simulink library "Dequiv"  (Simulink 3.00)
settings Model: LastModifiedBy=campa

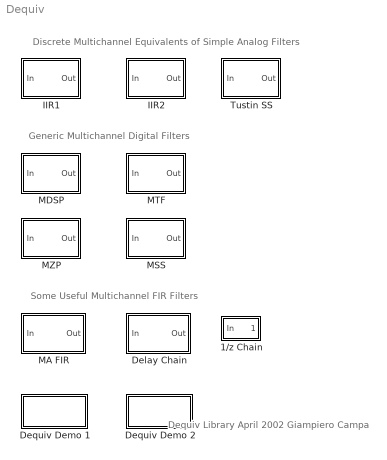
== system Dequiv ==
  note: Discrete Multichannel Equivalents of Simple Analog Filters
  note: Some Useful Multichannel FIR Filters
  note: Dequiv Library
      | April 2002
      | Giampiero Campa
  note: Generic Multichannel Digital Filters
  1/z Chain : Subsystem  mask(Discrete Time FIFO Chain){ni=1, rd=4, x0=0, T=0.025}
      mask prompts: ni "Number of Channels"; rd "Number of Delays for each Channel"; x0 "Initial Conditon"; T "Sample Time"
      mask help: Discrete Time FIFO Chain
      mask init:
      | a=[];b=[];c=[];d=[];
      | for i=1:ni,
      | a=[a,zeros(size(a,1),rd);zeros(rd,size(a,2)),diag(ones(rd-1,1),1)];
      | b=[b,zeros(size(b,1),1);zeros(rd,size(b,2)),[zeros(rd-1,1);1]];
      | c=[c,zeros(size(c,1),rd);zeros(1,size(c,2)),[1 zeros(1,rd-1)]];
      | d=[d,zeros(size(d,1),1);zeros(1,size(d,2)),0];
      | end
      mask Help: Discrete Time FIFO Chain
      mask Display: disp('FIFO')
  Delay Chain : Subsystem  mask(Delay Chain){ni=1, rd=3, x0=2e-7/4, T=0.025}
      mask prompts: ni "Number of Channels"; rd "Number of Delays"; x0 "Initial Condition"; T "Sample Time"
      mask help:
      | Implements a delay chain,
      |   each input is delayed n times and the respective
      |   outputs are all the states as well as the input itself.
      mask init:
      | a=[];b=[];c=[];d=[];
      | for i=1:ni,
      | a=[a,zeros(size(a,1),rd);zeros(rd,size(a,2)),diag(ones(rd-1,1),1)];
      | b=[b,zeros(size(b,1),1);zeros(rd,size(b,2)),[zeros(rd-1,1);1]];
      | c=[c,zeros(size(c,1),rd);zeros(rd+1,size(c,2)),[eye(rd);zeros(1,rd)]];
      | d=[d,zeros(size(d,1),1);zeros(rd+1,size(d,2)),[zeros(rd,1);1]];
      | end
      mask Help:
      | <p>
      | This block implements a MIMO Delay chain.
      | </p>
      | <p>
      |   The initial condition is for the whole system.
      |    If the input is an m-channel vector u, being u0 at time zero,
      |    and n is the number of delays, then a suitable initial condition is :
      |    x0=ones(n,1)*reshape(u0,1,m)
      | </p>
      mask Display: dpoly('1','z^n','')
  Dequiv Demo 1 : Subsystem
      settings: OpenFcn=digflt
      mask Display: disp('Example 1')
  Dequiv Demo 2 : Subsystem
      settings: OpenFcn=multifil;
      mask Display: disp('Example 2')
  IIR1 : Subsystem  mask(Discrete Time First Order IIR){ni=1, a=0.1, x0=0, T=0.025}
      mask prompts: ni "Number of Channels"; a "Cutoff Frequency (a)"; x0 "Initial Condition"; T "Sample Time"
      mask help:
      | Each channel has the transfer function
      |   (1-exp(-aT))/(1-exp(-aT)(z^-1)) which is a good
      |   (pz-matched) approximation of a/(s+a) if 10*a*T<pi
      mask init:
      | A=[];B=[];C=[];D=[];
      | for i=1:ni,
      | A=[A,zeros(size(A,1),1);zeros(1,size(A,2)),exp(-a*T)];
      | B=[B,zeros(size(B,1),1);zeros(1,size(B,2)),1-exp(-a*T)];
      | C=[C,zeros(size(C,1),1);zeros(1,size(C,2)),exp(-a*T)];
      | D=[D,zeros(size(D,1),1);zeros(1,size(D,2)),1-exp(-a*T)];
      | end
      mask Help:
      | <p>
      |   Each channel has the transfer function
      |   (1-exp(-aT))/(1-exp(-aT)(z^-1)) which is a good
      |   (pz-matched) approximation of a/(s+a) if 10*a*T<pi
      | </p>
      mask Display: dpoly(a,[1 a],'s')
  IIR2 : Subsystem  mask(Discrete Time Second Order IIR){ni=1, w=3, x=0.5, x0=0, T=0.025}
      mask prompts: ni "Number of Channels"; w "Poles Magnitude (m)"; x "Poles Damping (x)"; x0 "Initial Condition"; T "Sample Time"
      mask help:
      | Each channel has the transfer function :
      |   1-2*cos(sqrt(1-x^2)*m*T)*exp(-x*m*T)+exp(-2*x*m*T) /
      |   1-2*cos(sqrt(1-x^2)*m*T)*exp(-x*m*T)z^-1+exp(-2*x*m*T)z^-2
      |   which is a good (pz-matched) approximation of
      |   m^2/(s^2+2xms+m^2) if 10*m*T<pi
      |   The initial condition is in discrete time for the whole system.
      mask init:
      | A=[];B=[];C=[];D=[];
      | for i=1:ni,
      | A=[A,zeros(size(A,1),2);zeros(2,size(A,2)),[0 1; -exp(-2*x*w*T) 2*cos(sqrt(1-x^2)*w*T)*exp(-x*w*T)]];
      | B=[B,zeros(size(B,1),1);zeros(2,size(B,2)),[0;1+exp(-2*x*w*T)-2*cos(sqrt(1-x^2)*w*T)*exp(-x*w*T)]];
      | C=[C,zeros(size(C,1),2);zeros(1,size(C,2)),[-exp(-2*x*w*T)  2*cos(sqrt(1-x^2)*w*T)*exp(-x*w*T)]];
      | D=[D,zeros(size(D,1),1);zeros(1,size(D,2)),1+exp(-2*x*w*T)-2*cos(sqrt(1-x^2)*w*T)*exp(-x*w*T)];
      | end
      mask Help:
      | <p>
      |   Each channel has the transfer function :
      |   1-2*cos(sqrt(1-x^2)*m*T)*exp(-x*m*T)+exp(-2*x*m*T) /
      |   1-2*cos(sqrt(1-x^2)*m*T)*exp(-x*m*T)z^-1+exp(-2*x*m*T)z^-2
      |   which is a good (pz-matched) approximation of
      |   m^2/(s^2+2xms+m^2) if 10*m*T<pi
      | </p>
      | <p>
      |   The initial condition is in discrete time for the whole system.
      |    If the input is an m-channel vector u, being u0 at time zero,
      |    then a suitable initial condition is : x0=ones(2,1)*reshape(u0,1,m)
      | </p>
      mask Display: dpoly(w^2, [1 2*x*w w^2],'s')
  MA FIR : Subsystem  mask(Discrete Time Moving Average FIR){ni=1, ws=50, x0=2e-7/4, T=0.025}
      mask prompts: ni "Number of Channels"; ws "Window Size"; x0 "Initial Condition"; T "Sample Time"
      mask help: Discrete Time Moving Average FIR
      mask init:
      | a=[];b=[];c=[];d=[];rd=ws-1;
      | for i=1:ni,
      | a=[a,zeros(size(a,1),rd);zeros(rd,size(a,2)),diag(ones(rd-1,1),1)];
      | b=[b,zeros(size(b,1),1);zeros(rd,size(b,2)),[zeros(rd-1,1);1]];
      | c=[c,zeros(size(c,1),rd);zeros(1,size(c,2)),[ones(1,rd)/(rd+1)]];
      | d=[d,zeros(size(d,1),1);zeros(1,size(d,2)),1/(rd+1)];
      | end
      mask Help:
      | <p>
      | This block implements a MIMO Discrete Time Moving Average FIR.
      | </p>
      | <p>
      |   The initial condition is or the whole system.
      |    If the input is an m-channel vector u, being u0 at time zero,
      |    and ord is the maximum power of z, (ord=length(num)-1)
      |    then a suitable initial condition is : x0=ones(ord,1)*reshape(u0,1,m)
      | </p>
      mask Display: dpoly('1+z+z^2+..','z^n','')
  MDSP : Subsystem  mask(Generic Multichannel Digital Filter (DSP Convention)){ni=1, num=[1 0], den=[1 0.5], u0=0, T=0.025}
      mask prompts: ni "Number of Channels"; num "num (ascending powers of z^-1)"; den "den (ascending powers of z^-1)"; u0 "Initial input (for the whole system)"; T "Sample Time"
      mask help:
      | Each channel has the transfer function num/den
      |   where num and den contains coefficients of z^-1
      |   in ascending order (DSP convention).
      |   See also the file tf.m for more info about the DSP convention.
      |   The initial state is set for the whole system as the steady state
      |   value corresponding to the given input.
      mask init:
      | [a,b,c,d]=ssdata(ss(tf(num,den,T,'Variable','z^-1')));
      | A=[];B=[];C=[];D=[];
      | for i=1:ni,
      | A=[A,zeros(size(A,1),size(a,2));zeros(size(a,1),size(A,2)),a];
      | B=[B,zeros(size(B,1),size(b,2));zeros(size(b,1),size(B,2)),b];
      | C=[C,zeros(size(C,1),size(c,2));zeros(size(c,1),size(C,2)),c];
      | D=[D,zeros(size(D,1),size(d,2));zeros(size(d,1),size(D,2)),d];
      | end
      | if max(size(u0))==1, u0=ones(size(B,2),1)*u0; end
      | x0=pinv(eye(size(A))-A)*B*u0;
      mask Help:
      | <p>
      |   Each channel has the transfer function num/den
      |   where num and den contains coefficients of z^-1
      |   in ascending order (DSP convention).
      |   See also the file tf.m for more info about the DSP convention.
      | </p>
      | <p>
      |   The initial state is set for the whole system as the steady state
      |   value corresponding to the given input. That is x0=inv(I-A)*B*u0
      |   where A,B,u0 are representative of the whole system.
      | </p>
      mask Display: dpoly(num,den,'z-1')
  MSS : Subsystem  mask(Multichannel Discrete State Space){n=1, a=[0 1;-3^2 -2*3*0.74], b=[0;3^2], c=[1 0], d=0, u0=0, T=0.025}
      mask prompts: n "Number of Blocks"; u0 "Initial input (for the whole system)"; T "Sample Time"
      mask help:
      | The resulting system is the diagonal composition of n blocks.
      |   Each block consists in the MIMO discrete time state space
      |   system A,B,C,D.
      |   The initial state is set for the whole system as the steady state
      |   value corresponding to the given input.
      mask init:
      | A=[];B=[];C=[];D=[];
      | for i=1:n,
      | A=[A,zeros(size(A,1),size(a,2));zeros(size(a,1),size(A,2)),a];
      | B=[B,zeros(size(B,1),size(b,2));zeros(size(b,1),size(B,2)),b];
      | C=[C,zeros(size(C,1),size(c,2));zeros(size(c,1),size(C,2)),c];
      | D=[D,zeros(size(D,1),size(d,2));zeros(size(d,1),size(D,2)),d];
      | end
      | if max(size(u0))==1, u0=ones(size(B,2),1)*u0; end
      | x0=pinv(eye(size(A))-A)*B*u0;
      mask Help:
      | <p>
      |   The resulting system is the diagonal composition of n blocks.
      |   Each block consists in the MIMO discrete time state space
      |   system A,B,C,D.
      | </p>
      | <p>
      |   The initial state is set for the whole system as the steady state
      |   value corresponding to the given input. That is x0=inv(I-A)*B*u0
      |   where A,B,u0 are representative of the whole system.
      | </p>
      mask Display: fprintf('x+ = Ax + Bu\n  y = Cx + Du');
  MTF : Subsystem  mask(Generic Multichannel Transfer Function){ni=1, num=[1 0], den=[1 0.5], u0=0, T=0.025}
      mask prompts: ni "Number of Channels"; num "num (descending powers of z)"; den "den (descending powers of z)"; u0 "Initial input"; T "Sample Time"
      mask help:
      | Each channel has the transfer function num/den
      |   where num and den contains coefficients of z
      |   in descending order (TF convention).
      |   See also the file tf.m for more info about the TF convention.
      |   The initial state is set for the whole system as the steady state
      |   value corresponding to the given input.
      mask init:
      | [a,b,c,d]=ssdata(ss(tf(num,den,T)));
      | A=[];B=[];C=[];D=[];
      | for i=1:ni,
      | A=[A,zeros(size(A,1),size(a,2));zeros(size(a,1),size(A,2)),a];
      | B=[B,zeros(size(B,1),size(b,2));zeros(size(b,1),size(B,2)),b];
      | C=[C,zeros(size(C,1),size(c,2));zeros(size(c,1),size(C,2)),c];
      | D=[D,zeros(size(D,1),size(d,2));zeros(size(d,1),size(D,2)),d];
      | end
      | if max(size(u0))==1, u0=ones(size(B,2),1)*u0; end
      | x0=pinv(eye(size(A))-A)*B*u0;
      mask Help:
      | <p>
      |   Each channel has the transfer function num/den
      |   where num and den contains coefficients of z
      |   in ascending order (TF convention).
      |   See also the file tf.m for more info about the DSP convention.
      | </p>
      | <p>
      |   The initial state is set for the whole system as the steady state
      |   value corresponding to the given input. That is x0=inv(I-A)*B*u0
      |   where A,B,u0 are representative of the whole system.
      | </p>
      mask Display: dpoly(num,den,'z')
  MZP : Subsystem  mask(Generic Multichannel Zero-Pole){ni=1, Z=[1 0], P=[1 0.5], K=1, u0=0, T=0.025}
      mask prompts: ni "Number of Channels"; Z "zeros"; P "poles"; K "gain"; u0 "Initial input (for the whole system)"; T "Sample Time"
      mask help:
      | Each channel has the transfer function num/den
      |   where num and den are calculated from the zeros,
      |   poles and gain entered in the mask.
      |   See also the file zpk.m for more info about the ZPK convention.
      |   The initial state is set for the whole system as the steady state
      |   value corresponding to the given input.
      mask init:
      | [a,b,c,d]=ssdata(ss(zpk(Z,P,K,T)));
      | A=[];B=[];C=[];D=[];
      | for i=1:ni,
      | A=[A,zeros(size(A,1),size(a,2));zeros(size(a,1),size(A,2)),a];
      | B=[B,zeros(size(B,1),size(b,2));zeros(size(b,1),size(B,2)),b];
      | C=[C,zeros(size(C,1),size(c,2));zeros(size(c,1),size(C,2)),c];
      | D=[D,zeros(size(D,1),size(d,2));zeros(size(d,1),size(D,2)),d];
      | end
      | if max(size(u0))==1, u0=ones(size(B,2),1)*u0; end
      | x0=pinv(eye(size(A))-A)*B*u0;
      mask Help:
      | <p>
      |   Each channel has the transfer function num/den
      |   where num and den are calculated from the zeros,
      |   poles and gain entered in the mask.
      |   See also the file zpk.m for more info about the ZPK convention.
      | </p>
      | <p>
      |   The initial state is set for the whole system as the steady state
      |   value corresponding to the given input. That is x0=inv(I-A)*B*u0
      |   where A,B,u0 are representative of the whole system.
      | </p>
      mask Display: droots(Z,P,K,'z')
  Tustin SS : Subsystem  mask(Tustin Approximation of Continuous State Space){n=1, a=[0 1;-3^2 -2*3*0.74], b=[0;3^2], c=[1 0], d=0, w=1, u0=0, T=0.025}
      mask prompts: n "Number of Blocks"; w "Prewarping (w<pi/T, w=0 for bilinear approx)"; u0 "Initial Input"; T "Sample Time"
      mask help:
      | The resulting system is the diagonal composition of n blocks.
      |   Each block consists in the discrete time Tustin approximation
      |   of the MIMO continuous time state space system A,B,C,D.
      |   The initial condition is set for the whole system as the steady state
      |   discrete-time value corresponding to the given input.
      mask init:
      | if abs(w)<1e-15, h=T; else h=2/w*tan(w*T/2); end
      | I=eye(size(a));X=inv(I-a*h/2);
      | A=[];B=[];C=[];D=[];
      | for i=1:n,
      | A=[A,zeros(size(A,1),size(a,2));zeros(size(a,1),size(A,2)),X*(I+a*h/2)];
      | B=[B,zeros(size(B,1),size(b,2));zeros(size(b,1),size(B,2)),sqrt(h)*X*b];
      | C=[C,zeros(size(C,1),size(c,2));zeros(size(c,1),size(C,2)),sqrt(h)*c*X];
      | D=[D,zeros(size(D,1),size(d,2));zeros(size(d,1),size(D,2)),d+c*X*b*h/2];
      | end
      | if max(size(u0))==1, u0=ones(size(B,2),1)*u0; end
      | x0=pinv(eye(size(A))-A)*B*u0;
      mask Help:
      | <p>
      |   The resulting system is the diagonal composition of n blocks.
      |   Each block consists in the discrete time Tustin approximation
      |   of the MIMO continuous time state space system A,B,C,D.
      | </p>
      | <p>
      |   The initial state is set for the whole system as the steady state
      |   value corresponding to the given input. That is x0=inv(I-A)*B*u0
      |   where A,B,u0 are representative of the whole system.
      | </p>
      mask Display: disp('Tustin')

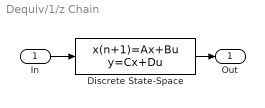
== system Dequiv/1/z Chain ==
  In : Inport  Port=1  PortWidth=-1  SampleTime=-1  DataType=auto
      settings: SignalType=auto
  Discrete State-Space : DiscreteStateSpace  A=a  B=b  C=c  D=d  X0=x0  SampleTime=T
  Out : Outport  Port=1
  wires:
  Discrete State-Space/1 -> Out/1
  In/1 -> Discrete State-Space/1

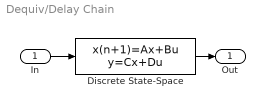
== system Dequiv/Delay Chain ==
  In : Inport  Port=1  PortWidth=-1  SampleTime=-1  DataType=auto
      settings: SignalType=auto
  Discrete State-Space : DiscreteStateSpace  A=a  B=b  C=c  D=d  X0=x0  SampleTime=T
  Out : Outport  Port=1
  wires:
  Discrete State-Space/1 -> Out/1
  In/1 -> Discrete State-Space/1

== system Dequiv/Dequiv Demo 1 ==

== system Dequiv/Dequiv Demo 2 ==

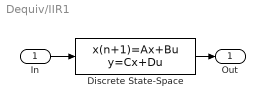
== system Dequiv/IIR1 ==
  In : Inport  Port=1  PortWidth=-1  SampleTime=-1  DataType=auto
      settings: SignalType=auto
  Discrete State-Space : DiscreteStateSpace  A=A  B=B  C=C  D=D  X0=x0  SampleTime=T
  Out : Outport  Port=1
  wires:
  In/1 -> Discrete State-Space/1
  Discrete State-Space/1 -> Out/1

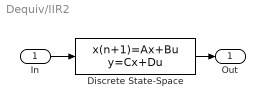
== system Dequiv/IIR2 ==
  In : Inport  Port=1  PortWidth=-1  SampleTime=-1  DataType=auto
      settings: SignalType=auto
  Discrete State-Space : DiscreteStateSpace  A=A  B=B  C=C  D=D  X0=x0  SampleTime=T
  Out : Outport  Port=1
  wires:
  Discrete State-Space/1 -> Out/1
  In/1 -> Discrete State-Space/1

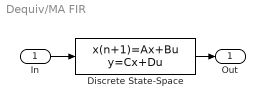
== system Dequiv/MA FIR ==
  In : Inport  Port=1  PortWidth=-1  SampleTime=-1  DataType=auto
      settings: SignalType=auto
  Discrete State-Space : DiscreteStateSpace  A=a  B=b  C=c  D=d  X0=x0  SampleTime=T
  Out : Outport  Port=1
  wires:
  In/1 -> Discrete State-Space/1
  Discrete State-Space/1 -> Out/1

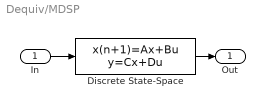
== system Dequiv/MDSP ==
  In : Inport  Port=1  PortWidth=-1  SampleTime=-1  DataType=auto
      settings: SignalType=auto
  Discrete State-Space : DiscreteStateSpace  A=A  B=B  C=C  D=D  X0=x0  SampleTime=T
  Out : Outport  Port=1
  wires:
  In/1 -> Discrete State-Space/1
  Discrete State-Space/1 -> Out/1

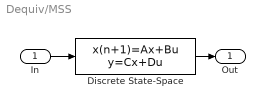
== system Dequiv/MSS ==
  In : Inport  Port=1  PortWidth=-1  SampleTime=-1  DataType=auto
      settings: SignalType=auto
  Discrete State-Space : DiscreteStateSpace  A=A  B=B  C=C  D=D  X0=x0  SampleTime=T
  Out : Outport  Port=1
  wires:
  Discrete State-Space/1 -> Out/1
  In/1 -> Discrete State-Space/1

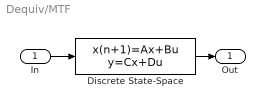
== system Dequiv/MTF ==
  In : Inport  Port=1  PortWidth=-1  SampleTime=-1  DataType=auto
      settings: SignalType=auto
  Discrete State-Space : DiscreteStateSpace  A=A  B=B  C=C  D=D  X0=x0  SampleTime=T
  Out : Outport  Port=1
  wires:
  Discrete State-Space/1 -> Out/1
  In/1 -> Discrete State-Space/1

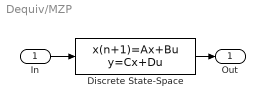
== system Dequiv/MZP ==
  In : Inport  Port=1  PortWidth=-1  SampleTime=-1  DataType=auto
      settings: SignalType=auto
  Discrete State-Space : DiscreteStateSpace  A=A  B=B  C=C  D=D  X0=x0  SampleTime=T
  Out : Outport  Port=1
  wires:
  In/1 -> Discrete State-Space/1
  Discrete State-Space/1 -> Out/1

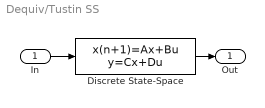
== system Dequiv/Tustin SS ==
  In : Inport  Port=1  PortWidth=-1  SampleTime=-1  DataType=auto
      settings: SignalType=auto
  Discrete State-Space : DiscreteStateSpace  A=A  B=B  C=C  D=D  X0=x0  SampleTime=T
  Out : Outport  Port=1
  wires:
  In/1 -> Discrete State-Space/1
  Discrete State-Space/1 -> Out/1
